simulink model "state"  (Simulink 7.9)
settings: Solver=ode45  StartTime=0.0  StopTime=6  RelTol=1e-3
libraries: simulink x1
settings Model: Creator=zhuye  LastModifiedBy=lzc
settings DebuggingCC: SolverPrmCheckMsg=none  ParameterPrecisionLossMsg=none

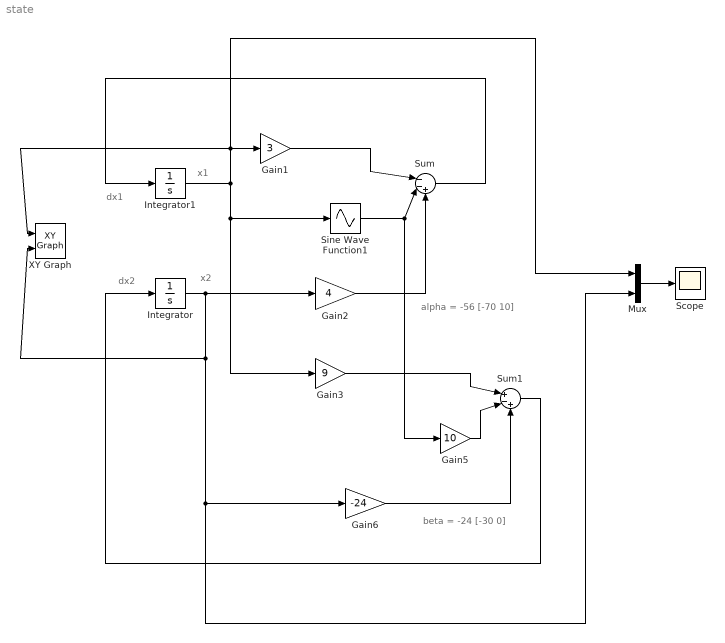
== system state ==
  note: x1
  note: x2
  note: dx1
  note: dx2
  note: alpha = -56 [-70 10]
  note: beta = -24 [-30 0]
  Gain1 : Gain  Gain=3
  Gain2 : Gain  Gain=4
  Gain3 : Gain  Gain=9
  Gain5 : Gain  Gain=10
  Gain6 : Gain  Gain=-24
  Integrator : Integrator  InitialCondition=80
  Integrator1 : Integrator  InitialCondition=-80
  Mux : Mux  Inputs=2
  Scope : Scope
  Sine Wave Function1 : Sin  TimeSource=Use external signal  SampleTime=0
  Sum : Sum  Inputs=|--+
  Sum1 : Sum  Inputs=|+-+
  XY Graph : simulink/Sinks/XY Graph  xmin=-200  xmax=160  ymin=-80  ymax=100  st=-1
  wires:
  Integrator1/1 -> Gain3/1, Sine Wave Function1/1, Gain1/1, XY Graph/1, Mux/1
  Gain1/1 -> Sum/1
  Sine Wave Function1/1 -> Sum/2, Gain5/1
  Integrator/1 -> Gain2/1, XY Graph/2, Gain6/1, Mux/2
  Gain2/1 -> Sum/3
  Gain3/1 -> Sum1/1
  Gain5/1 -> Sum1/2
  Gain6/1 -> Sum1/3
  Sum/1 -> Integrator1/1
  Sum1/1 -> Integrator/1
  Mux/1 -> Scope/1
